simulink model "ex_5"  (R2014a)
settings: Solver=ode45  StartTime=0.0  StopTime=10.0  RelTol=1e-3
settings Model: Creator=Pedro  LastModifiedBy=samuel
settings DebuggingCC: MergeDetectMultiDrivingBlocksExec=error

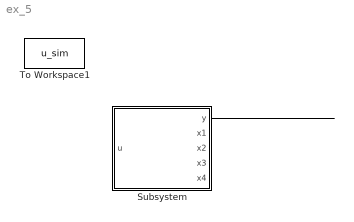
== system ex_5 ==
  Subsystem : Subsystem
  To Workspace1 : ToWorkspace  VariableName=u_sim  SaveFormat=Timeseries  SampleTime=-1
  wires:
  ? -> To Workspace1/1, Subsystem/1(u)
  Subsystem/1(y) -> ?

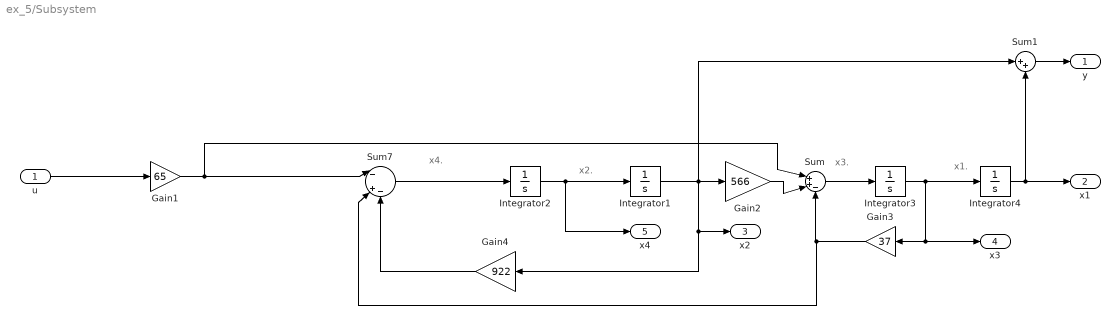
== system ex_5/Subsystem ==
  note: x1.
  note: x3.
  note: x2.
  note: x4.
  u : Inport
  Gain1 : Gain  Gain=65
  Gain2 : Gain  Gain=566
  Gain3 : Gain  Gain=37
  Gain4 : Gain  Gain=922
  Integrator{1..4} (4 alike) : Integrator
  Sum : Sum  Inputs=|++-
  Sum1 : Sum  Inputs=|++
  Sum7 : Sum  Inputs=|-|+-
  y : Outport
  x1 : Outport  Port=2
  x2 : Outport  Port=3
  x3 : Outport  Port=4
  x4 : Outport  Port=5
  wires:
  Sum7/1 -> Integrator2/1
  Integrator2/1 -> Integrator1/1, x4/1
  Gain1/1 -> Sum/1, Sum7/1
  u/1 -> Gain1/1
  Integrator1/1 -> Gain4/1, x2/1, Sum1/1, Gain2/1
  Sum/1 -> Integrator3/1
  Gain2/1 -> Sum/2
  Integrator3/1 -> Integrator4/1, x3/1, Gain3/1
  Gain3/1 -> Sum7/2, Sum/3
  Integrator4/1 -> x1/1, Sum1/2
  Gain4/1 -> Sum7/3
  Sum1/1 -> y/1
